simulink library "NullHardware"  (R2014a)
settings: Solver=ode45  SolverMode=SingleTasking  StartTime=0.0  StopTime=10.0  RelTol=1e-3
settings Model: Creator=cbeal  LastModifiedBy=cbeal

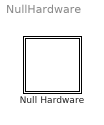
== system NullHardware ==
  Null Hardware : Subsystem
      mask Display: disp('-0-');

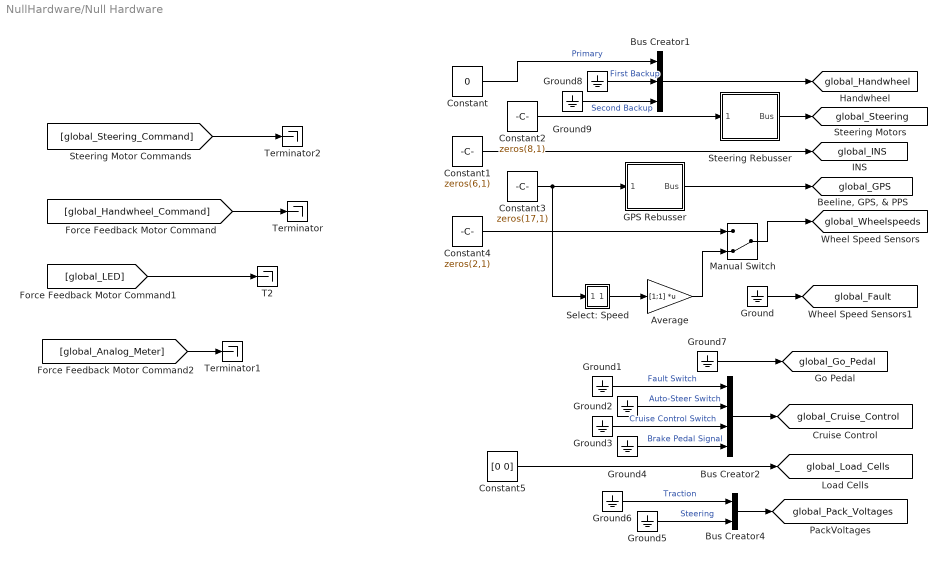
== system NullHardware/Null Hardware ==
  Average : Gain  Gain=[1;1]  Multiplication=Matrix(K*u)  SaturateOnIntegerOverflow=on  OutDataTypeStr=Inherit: Same as input  ParamDataTypeStr=Inherit: Same as input
  Bus Creator1 : BusCreator  Inputs=3
  Bus Creator2 : BusCreator
  Bus Creator4 : BusCreator  Inputs=2
  Constant : Constant  Value=0
  Constant1 : Constant  Value=zeros(6,1)
  Constant2 : Constant  Value=zeros(8,1)
  Constant3 : Constant  Value=zeros(17,1)
  Constant4 : Constant  Value=zeros(2,1)
  Constant5 : Constant  Value=[0 0]
  GPS Rebusser : Subsystem
  Ground{,1..9} (10 alike) : Ground
  Manual Switch : ManualSwitch  CurrentSetting=0
  Select: Speed : Subsystem  mask{indices=13, width=17}
      mask prompts: indices "Signal indices"; width "Input width"
      mask init:
      | ic=length(indices);
      | 
      | K=zeros(ic,width);
      | 
      | for ii=1:ic,
      | 	K(ii,indices(ii))=1;
      | end
      mask Display: disp(indices)
  Steering Rebusser : Subsystem
  T2 : Terminator
  Terminator : Terminator
  Terminator1 : Terminator
  Terminator2 : Terminator
  tag scope: global_Cruise_Control=global, global_Fault=global, global_GPS=global, global_Go_Pedal=global, global_Handwheel=global, global_INS=global, global_Load_Cells=global, global_Pack_Voltages=global, global_Steering=global, global_Wheelspeeds=global
  wires:
  Ground7/1 -> [global_Go_Pedal]
  Ground6/1 -> Bus Creator4/1  "Traction"
  Bus Creator4/1 -> [global_Pack_Voltages]
  Ground5/1 -> Bus Creator4/2  "Steering"
  Ground4/1 -> Bus Creator2/4  "Brake Pedal Signal"
  Ground3/1 -> Bus Creator2/3  "Cruise Control Switch"
  Ground2/1 -> Bus Creator2/2  "Auto-Steer Switch"
  Ground1/1 -> Bus Creator2/1  "Fault Switch"
  Bus Creator2/1 -> [global_Cruise_Control]
  Constant2/1 -> Steering Rebusser/1(Vector)
  Average/1 -> Manual Switch/2
  Constant4/1 -> Manual Switch/1
  Manual Switch/1 -> [global_Wheelspeeds]
  Select: Speed/1(Out1) -> Average/1
  Constant3/1 -> Select: Speed/1(In1), GPS Rebusser/1(Vector)
  GPS Rebusser/1(Bus) -> [global_GPS]
  Steering Rebusser/1(Bus) -> [global_Steering]
  [global_LED] -> T2/1
  Ground/1 -> [global_Fault]
  Constant1/1 -> [global_INS]
  [global_Handwheel_Command] -> Terminator/1
  [global_Steering_Command] -> Terminator2/1
  [global_Analog_Meter] -> Terminator1/1
  Constant5/1 -> [global_Load_Cells]
  Bus Creator1/1 -> [global_Handwheel]
  Constant/1 -> Bus Creator1/1  "Primary"
  Ground8/1 -> Bus Creator1/2  "First Backup"
  Ground9/1 -> Bus Creator1/3  "Second Backup"

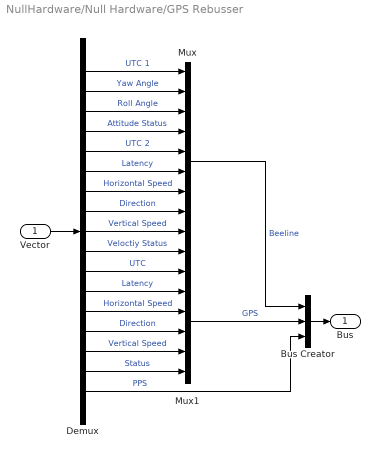
== system NullHardware/Null Hardware/GPS Rebusser ==
  Vector : Inport
  Bus Creator : BusCreator  Inputs=3
  Demux : Demux  Outputs=17
  Mux : Mux  Inputs=10
  Mux1 : Mux  Inputs=6
  Bus : Outport
  wires:
  Mux/1 -> Bus Creator/1  "Beeline"
  Demux/10 -> Mux/10  "Veloctiy Status"
  Demux/9 -> Mux/9  "Vertical Speed"
  Demux/8 -> Mux/8  "Direction"
  Demux/7 -> Mux/7  "Horizontal Speed"
  Demux/6 -> Mux/6  "Latency"
  Demux/5 -> Mux/5  "UTC 2"
  Demux/4 -> Mux/4  "Attitude Status"
  Demux/3 -> Mux/3  "Roll Angle"
  Demux/2 -> Mux/2  "Yaw Angle"
  Demux/1 -> Mux/1  "UTC 1"
  Mux1/1 -> Bus Creator/2  "GPS"
  Demux/16 -> Mux1/6  "Status"
  Demux/15 -> Mux1/5  "Vertical Speed"
  Demux/14 -> Mux1/4  "Direction"
  Demux/13 -> Mux1/3  "Horizontal Speed"
  Demux/12 -> Mux1/2  "Latency"
  Demux/11 -> Mux1/1  "UTC"
  Demux/17 -> Bus Creator/3  "PPS"
  Vector/1 -> Demux/1
  Bus Creator/1 -> Bus/1

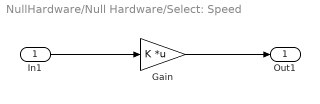
== system NullHardware/Null Hardware/Select: Speed ==
  In1 : Inport
  Gain : Gain  Gain=K  Multiplication=Matrix(K*u)  SaturateOnIntegerOverflow=on  OutDataTypeStr=Inherit: Same as input  ParamDataTypeStr=Inherit: Same as input
  Out1 : Outport
  wires:
  In1/1 -> Gain/1
  Gain/1 -> Out1/1

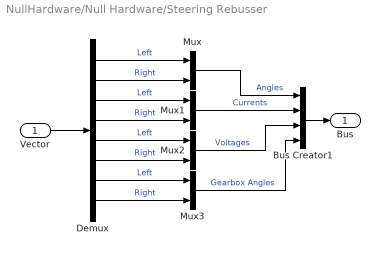
== system NullHardware/Null Hardware/Steering Rebusser ==
  Vector : Inport
  Bus Creator1 : BusCreator
  Demux : Demux  Outputs=8
  Mux{,1..3} (4 alike) : Mux  Inputs=2
  Bus : Outport
  wires:
  Mux2/1 -> Bus Creator1/3  "Voltages"
  Mux1/1 -> Bus Creator1/2  "Currents"
  Mux/1 -> Bus Creator1/1  "Angles"
  Demux/6 -> Mux2/2  "Right"
  Demux/5 -> Mux2/1  "Left"
  Demux/4 -> Mux1/2  "Right"
  Demux/3 -> Mux1/1  "Left"
  Demux/2 -> Mux/2  "Right"
  Demux/1 -> Mux/1  "Left"
  Vector/1 -> Demux/1
  Bus Creator1/1 -> Bus/1
  Mux3/1 -> Bus Creator1/4  "Gearbox Angles"
  Demux/7 -> Mux3/1  "Left"
  Demux/8 -> Mux3/2  "Right"
